simulink model "SF015A_WhlImbRejctn"  (R2013b)
settings: Solver=FixedStepDiscrete  SolverMode=SingleTasking  StartTime=0.0  StopTime=1  FixedStep=0.002  RelTol=1e-3
values from neighbouring files (symbols this model uses):
  ACTIVBANDMAX_ULS_U32 = DataDict.Constant    [SF015A_WhlImbRejctn_DataDict.m]
  ADAPVFILMAX_ULS_F32 = DataDict.Constant    [SF015A_WhlImbRejctn_DataDict.m]
  ARCHGLBPRM_180OVERPI_ULS_F32 = DataDict.Constant    [SF015A_WhlImbRejctn_DataDict.m]
  ARCHGLBPRM_2MILLISEC_SEC_F32 = DataDict.Constant    [SF015A_WhlImbRejctn_DataDict.m]
  ARCHGLBPRM_2PI_ULS_F32 = DataDict.Constant    [SF015A_WhlImbRejctn_DataDict.m]
  ARCHGLBPRM_FLOATZEROTHD_ULS_F32 = DataDict.Constant    [SF015A_WhlImbRejctn_DataDict.m]
  ARCHGLBPRM_PI_ULS_F32 = DataDict.Constant    [SF015A_WhlImbRejctn_DataDict.m]
  ARCHGLBPRM_PIOVER180_ULS_F32 = DataDict.Constant    [SF015A_WhlImbRejctn_DataDict.m]
  ARCHGLBPRM_PIOVER2_ULS_F32 = DataDict.Constant    [SF015A_WhlImbRejctn_DataDict.m]
  CALMINSPERCOUNT_ULS_F32 = DataDict.Constant    [SF015A_WhlImbRejctn_DataDict.m]
  DURATIONDISABLE_CNT_U16 = DataDict.Constant    [SF015A_WhlImbRejctn_DataDict.m]
  FILTWHLSPDMAX_MOTRADPERSEC_F32 = DataDict.Constant    [SF015A_WhlImbRejctn_DataDict.m]
  MICROSECTOMILLISEC_ULS_F32 = DataDict.Constant    [SF015A_WhlImbRejctn_DataDict.m]
  MINSTOMILLISEC_ULS_F32 = DataDict.Constant    [SF015A_WhlImbRejctn_DataDict.m]
  NINETY_ULS_F32 = DataDict.Constant    [SF015A_WhlImbRejctn_DataDict.m]
  NODEBSTEP_CNT_U16 = DataDict.Constant    [SF015A_WhlImbRejctn_DataDict.m]
  NROFDLY_CNT_U08 = DataDict.Constant    [SF015A_WhlImbRejctn_DataDict.m]
  ONEHALF_ULS_F32 = DataDict.Constant    [SF015A_WhlImbRejctn_DataDict.m]
  ONEHUNDRED_ULS_F32 = DataDict.Constant    [SF015A_WhlImbRejctn_DataDict.m]
  ONEOVRTHREE_ULS_F32 = DataDict.Constant    [SF015A_WhlImbRejctn_DataDict.m]
  ONEOVRTWENTY_ULS_F32 = DataDict.Constant    [SF015A_WhlImbRejctn_DataDict.m]
  ONETHOUSAND_ULS_F32 = DataDict.Constant    [SF015A_WhlImbRejctn_DataDict.m]
  PEAKMAX_ULS_F32 = DataDict.Constant    [SF015A_WhlImbRejctn_DataDict.m]
  PEAKMIN_ULS_F32 = DataDict.Constant    [SF015A_WhlImbRejctn_DataDict.m]
  PHAADJMAX_ULS_F32 = DataDict.Constant    [SF015A_WhlImbRejctn_DataDict.m]
  PITIMESSAMPLETIME_ULS_F32 = DataDict.Constant    [SF015A_WhlImbRejctn_DataDict.m]
  STOREDMINSPERCOUNT_ULS_F32 = DataDict.Constant    [SF015A_WhlImbRejctn_DataDict.m]
  TWO_ULS_F32 = DataDict.Constant    [SF015A_WhlImbRejctn_DataDict.m]
  TWOOVRTHREE_ULS_F32 = DataDict.Constant    [SF015A_WhlImbRejctn_DataDict.m]
  WhlImbRejctnAdpvFac = DataDict.Calibration    [SF015A_WhlImbRejctn_DataDict.m]
  WhlImbRejctnAutScaEna = DataDict.Calibration    [SF015A_WhlImbRejctn_DataDict.m]
  WhlImbRejctnAutScaTar = DataDict.Calibration    [SF015A_WhlImbRejctn_DataDict.m]
  WhlImbRejctnCurrMgnSlewPerLoop = DataDict.Calibration    [SF015A_WhlImbRejctn_DataDict.m]
  WhlImbRejctnDcTrendFltRcvryDly = DataDict.Calibration    [SF015A_WhlImbRejctn_DataDict.m]
  WhlImbRejctnDcTrendFltRcvryNegStep = DataDict.Calibration    [SF015A_WhlImbRejctn_DataDict.m]
  WhlImbRejctnDcTrendFltRcvryPosStep = DataDict.Calibration    [SF015A_WhlImbRejctn_DataDict.m]
  WhlImbRejctnDcTrendFltRcvryThd = DataDict.Calibration    [SF015A_WhlImbRejctn_DataDict.m]
  WhlImbRejctnDcTrendTh2Tq = DataDict.Calibration    [SF015A_WhlImbRejctn_DataDict.m]
  WhlImbRejctnDcTrendThTq = DataDict.Calibration    [SF015A_WhlImbRejctn_DataDict.m]
  WhlImbRejctnDcTrendTi2Sec = DataDict.Calibration    [SF015A_WhlImbRejctn_DataDict.m]
  WhlImbRejctnDcTrendTiSec = DataDict.Calibration    [SF015A_WhlImbRejctn_DataDict.m]
  WhlImbRejctnEnaSlewPerLoop = DataDict.Calibration    [SF015A_WhlImbRejctn_DataDict.m]
  WhlImbRejctnFctEna = DataDict.Calibration    [SF015A_WhlImbRejctn_DataDict.m]
  WhlImbRejctnFrqDiagcAmpThd = DataDict.Calibration    [SF015A_WhlImbRejctn_DataDict.m]
  WhlImbRejctnFrqDiagcEna = DataDict.Calibration    [SF015A_WhlImbRejctn_DataDict.m]
  WhlImbRejctnFrqDiagcFltRcvryDly = DataDict.Calibration    [SF015A_WhlImbRejctn_DataDict.m]
  WhlImbRejctnFrqDiagcFltRcvryNegStep = DataDict.Calibration    [SF015A_WhlImbRejctn_DataDict.m]
  WhlImbRejctnFrqDiagcFltRcvryPosStep = DataDict.Calibration    [SF015A_WhlImbRejctn_DataDict.m]
  WhlImbRejctnFrqDiagcFltRcvryThd = DataDict.Calibration    [SF015A_WhlImbRejctn_DataDict.m]
  WhlImbRejctnFrqDiagcThd = DataDict.Calibration    [SF015A_WhlImbRejctn_DataDict.m]
  WhlImbRejctnFrqDiagcTout = DataDict.Calibration    [SF015A_WhlImbRejctn_DataDict.m]
  WhlImbRejctnFrqDiagcUgrPoleMgn = DataDict.Calibration    [SF015A_WhlImbRejctn_DataDict.m]
  WhlImbRejctnFrqScaTblX = DataDict.Calibration    [SF015A_WhlImbRejctn_DataDict.m]
  WhlImbRejctnMaxDurn = DataDict.Calibration    [SF015A_WhlImbRejctn_DataDict.m]
  WhlImbRejctnMaxMgn = DataDict.Calibration    [SF015A_WhlImbRejctn_DataDict.m]
  WhlImbRejctnMaxMgnFltNegStep = DataDict.Calibration    [SF015A_WhlImbRejctn_DataDict.m]
  WhlImbRejctnMaxMgnFltPosStep = DataDict.Calibration    [SF015A_WhlImbRejctn_DataDict.m]
  WhlImbRejctnMaxMgnFltRcvryDly = DataDict.Calibration    [SF015A_WhlImbRejctn_DataDict.m]
  WhlImbRejctnMaxMgnFltRcvryNegStep = DataDict.Calibration    [SF015A_WhlImbRejctn_DataDict.m]
  WhlImbRejctnMaxMgnFltRcvryPosStep = DataDict.Calibration    [SF015A_WhlImbRejctn_DataDict.m]
  WhlImbRejctnMaxMgnFltRcvryThd = DataDict.Calibration    [SF015A_WhlImbRejctn_DataDict.m]
  WhlImbRejctnMaxMgnFltThd = DataDict.Calibration    [SF015A_WhlImbRejctn_DataDict.m]
  WhlImbRejctnMgnEstimnDeltaSca = DataDict.Calibration    [SF015A_WhlImbRejctn_DataDict.m]
  WhlImbRejctnMgnEstimnDiThd = DataDict.Calibration    [SF015A_WhlImbRejctn_DataDict.m]
  WhlImbRejctnMgnEstimnEnaThd = DataDict.Calibration    [SF015A_WhlImbRejctn_DataDict.m]
  WhlImbRejctnMgnEstimnFrq = DataDict.Calibration    [SF015A_WhlImbRejctn_DataDict.m]
  WhlImbRejctnMgnEstimnFrqDelta = DataDict.Calibration    [SF015A_WhlImbRejctn_DataDict.m]
  WhlImbRejctnMgnEstimnLeak = DataDict.Calibration    [SF015A_WhlImbRejctn_DataDict.m]
  WhlImbRejctnRampDwnTi = DataDict.Calibration    [SF015A_WhlImbRejctn_DataDict.m]
  WhlImbRejctnScaCncl = DataDict.Calibration    [SF015A_WhlImbRejctn_DataDict.m]
  WhlImbRejctnUgrPoleMgn = DataDict.Calibration    [SF015A_WhlImbRejctn_DataDict.m]
  WhlImbRejctnVehSpdEna = DataDict.Calibration    [SF015A_WhlImbRejctn_DataDict.m]
  WhlImbRejctnWhlSpdCorrlnFltRcvryDly = DataDict.Calibration    [SF015A_WhlImbRejctn_DataDict.m]
  WhlImbRejctnWhlSpdCorrlnFltRcvryNegStep = DataDict.Calibration    [SF015A_WhlImbRejctn_DataDict.m]
  WhlImbRejctnWhlSpdCorrlnFltRcvryPosStep = DataDict.Calibration    [SF015A_WhlImbRejctn_DataDict.m]
  WhlImbRejctnWhlSpdCorrlnFltRcvryThd = DataDict.Calibration    [SF015A_WhlImbRejctn_DataDict.m]
  WhlImbRejctnWhlSpdCorrlnThd = DataDict.Calibration    [SF015A_WhlImbRejctn_DataDict.m]
  WhlImbRejctnWhlSpdCorrlnTi = DataDict.Calibration    [SF015A_WhlImbRejctn_DataDict.m]
  WIRCMDMAX_MOTNWTMTR_F32 = DataDict.Constant    [SF015A_WhlImbRejctn_DataDict.m]
  ZERO_ULS_F32 = DataDict.Constant    [SF015A_WhlImbRejctn_DataDict.m]
undefined symbols (not defined in the file or in its folder): Cntr, NtcNr1, NvmGetErrSts1, SigQlfr1, Sts, SysSt1
libraries: simulink x32, FixdToFloat x32, Fil x20, NxtrLim x15, NxtrNvM x12, NxtrAbslt x8, NxtrMath x7, NxtrMax x6, NxtrMin x4, FloatToFixd x2, LnrIntrpn x2, NxtrSign x1
(part 7 of 12)

== system SF015A_WhlImbRejctn/WhlImbRejctn/WhlImbRejctnPer1/WIR Diagnostics/DcTrendDiag/NoFault ==
  Input : Inport
  Action Port : ActionPort  ActionType=else
  CopyRight2 : Subsystem  Description=|  mask(Copyright Information){none=on}
      | Copyright info block.                                               
      |                                                                     
      | Place copyright information at the top of every subsystem in design.
      mask prompts: none "No parameters"
      mask help: Place copyright information at the top of every subsystem in design.
      mask Display:
      | NxtrConf = 'Nexteer Confidential';
      | 
      | sys = bdroot; %handle for the current model ("system")
      | first = get_param(sys,'Created');
      | if(isempty(first))
      |     first = datestr(now,'yyyy');
      | else
      |     first = first(end-3:end);  %year is last four digits
      | end
      | 
      | last = get_param(sys,'LastModifiedDate');
      | if isempty(last)
      |     last = datestr(now,'yyyy');
      | else
      |     last = last(end-3:end);
      | end
      | 
      | if strcmp(first,last)
      |     fprintf('%s -- Copyright %s Nexteer',NxtrConf,first)
      | else
      |     fprintf('%s -- %s%s- %s Nexteer',NxtrConf,char(169),first,last)
      | end
  Output : Outport
  wires:
  Input/1 -> Output/1

== system SF015A_WhlImbRejctn/WhlImbRejctn/WhlImbRejctnPer1/WIR Diagnostics/FrequencyDiag/CopyRight2 ==

== system SF015A_WhlImbRejctn/WhlImbRejctn/WhlImbRejctnPer1/WIR Diagnostics/FrequencyDiag/EnableDiag ==
  WIRCmdAmp : Inport
  FreqEst : Inport  Port=2
  WIRCmd : Inport  Port=3
  Enable : Inport  Port=4
  Action Port : ActionPort  ActionType=then
  CopyRight2 : Subsystem  Description=|  mask(Copyright Information){none=on}
      | Copyright info block.                                               
      |                                                                     
      | Place copyright information at the top of every subsystem in design.
      mask prompts: none "No parameters"
      mask help: Place copyright information at the top of every subsystem in design.
      mask Display:
      | NxtrConf = 'Nexteer Confidential';
      | 
      | sys = bdroot; %handle for the current model ("system")
      | first = get_param(sys,'Created');
      | if(isempty(first))
      |     first = datestr(now,'yyyy');
      | else
      |     first = first(end-3:end);  %year is last four digits
      | end
      | 
      | last = get_param(sys,'LastModifiedDate');
      | if isempty(last)
      |     last = datestr(now,'yyyy');
      | else
      |     last = last(end-3:end);
      | end
      | 
      | if strcmp(first,last)
      |     fprintf('%s -- Copyright %s Nexteer',NxtrConf,first)
      | else
      |     fprintf('%s -- %s%s- %s Nexteer',NxtrConf,char(169),first,last)
      | end
  Notch Comparison : Subsystem
  Output : Outport
  wires:
  Notch Comparison/1(FreqDiag) -> Output/1
  WIRCmdAmp/1 -> Notch Comparison/1(WIRCmdAmp)
  FreqEst/1 -> Notch Comparison/2(FreqEst)
  WIRCmd/1 -> Notch Comparison/3(WIRCmd)
  Enable/1 -> Notch Comparison/4(Enable)

== system SF015A_WhlImbRejctn/WhlImbRejctn/WhlImbRejctnPer1/WIR Diagnostics/FrequencyDiag/FreqDiagFault ==
  Input : Inport
  Action Port : ActionPort  ActionType=then
  CopyRight2 : Subsystem  Description=|  mask(Copyright Information){none=on}
      | Copyright info block.                                               
      |                                                                     
      | Place copyright information at the top of every subsystem in design.
      mask prompts: none "No parameters"
      mask help: Place copyright information at the top of every subsystem in design.
      mask Display:
      | NxtrConf = 'Nexteer Confidential';
      | 
      | sys = bdroot; %handle for the current model ("system")
      | first = get_param(sys,'Created');
      | if(isempty(first))
      |     first = datestr(now,'yyyy');
      | else
      |     first = first(end-3:end);  %year is last four digits
      | end
      | 
      | last = get_param(sys,'LastModifiedDate');
      | if isempty(last)
      |     last = datestr(now,'yyyy');
      | else
      |     last = last(end-3:end);
      | end
      | 
      | if strcmp(first,last)
      |     fprintf('%s -- Copyright %s Nexteer',NxtrConf,first)
      | else
      |     fprintf('%s -- %s%s- %s Nexteer',NxtrConf,char(169),first,last)
      | end
  Output : Outport
  wires:
  Input/1 -> Output/1

== system SF015A_WhlImbRejctn/WhlImbRejctn/WhlImbRejctnPer1/WIR Diagnostics/FrequencyDiag/NoDiag ==
  Input : Inport
  Action Port : ActionPort  ActionType=else
  CopyRight2 : Subsystem  Description=|  mask(Copyright Information){none=on}
      | Copyright info block.                                               
      |                                                                     
      | Place copyright information at the top of every subsystem in design.
      mask prompts: none "No parameters"
      mask help: Place copyright information at the top of every subsystem in design.
      mask Display:
      | NxtrConf = 'Nexteer Confidential';
      | 
      | sys = bdroot; %handle for the current model ("system")
      | first = get_param(sys,'Created');
      | if(isempty(first))
      |     first = datestr(now,'yyyy');
      | else
      |     first = first(end-3:end);  %year is last four digits
      | end
      | 
      | last = get_param(sys,'LastModifiedDate');
      | if isempty(last)
      |     last = datestr(now,'yyyy');
      | else
      |     last = last(end-3:end);
      | end
      | 
      | if strcmp(first,last)
      |     fprintf('%s -- Copyright %s Nexteer',NxtrConf,first)
      | else
      |     fprintf('%s -- %s%s- %s Nexteer',NxtrConf,char(169),first,last)
      | end
  Output : Outport
  wires:
  Input/1 -> Output/1

== system SF015A_WhlImbRejctn/WhlImbRejctn/WhlImbRejctnPer1/WIR Diagnostics/FrequencyDiag/NoFault ==
  Input : Inport
  Action Port : ActionPort  ActionType=else
  CopyRight2 : Subsystem  Description=|  mask(Copyright Information){none=on}
      | Copyright info block.                                               
      |                                                                     
      | Place copyright information at the top of every subsystem in design.
      mask prompts: none "No parameters"
      mask help: Place copyright information at the top of every subsystem in design.
      mask Display:
      | NxtrConf = 'Nexteer Confidential';
      | 
      | sys = bdroot; %handle for the current model ("system")
      | first = get_param(sys,'Created');
      | if(isempty(first))
      |     first = datestr(now,'yyyy');
      | else
      |     first = first(end-3:end);  %year is last four digits
      | end
      | 
      | last = get_param(sys,'LastModifiedDate');
      | if isempty(last)
      |     last = datestr(now,'yyyy');
      | else
      |     last = last(end-3:end);
      | end
      | 
      | if strcmp(first,last)
      |     fprintf('%s -- Copyright %s Nexteer',NxtrConf,first)
      | else
      |     fprintf('%s -- %s%s- %s Nexteer',NxtrConf,char(169),first,last)
      | end
  Output : Outport
  wires:
  Input/1 -> Output/1

== system SF015A_WhlImbRejctn/WhlImbRejctn/WhlImbRejctnPer1/WIR Diagnostics/MaxMagDiag/CopyRight2 ==

== system SF015A_WhlImbRejctn/WhlImbRejctn/WhlImbRejctnPer1/WIR Diagnostics/MaxMagDiag/Magnitude Comparison ==
  WIRCmdAmp1 : Inport
  Constant1 : Constant  Value=WhlImbRejctnMaxMgnFltPosStep
  Constant5 : Constant  Value=WhlImbRejctnMaxMgnFltNegStep
  Constant6 : Constant  Value=WhlImbRejctnMaxMgnFltThd
  Constant7 : Constant  Value=WhlImbRejctnMaxMgn
  CopyRight2 : Subsystem  Description=|  mask(Copyright Information){none=on}
      | Copyright info block.                                               
      |                                                                     
      | Place copyright information at the top of every subsystem in design.
      mask prompts: none "No parameters"
      mask help: Place copyright information at the top of every subsystem in design.
      mask Display:
      | NxtrConf = 'Nexteer Confidential';
      | 
      | sys = bdroot; %handle for the current model ("system")
      | first = get_param(sys,'Created');
      | first = first(end-3:end);  %year is last four digits
      | 
      | last = get_param(sys,'LastModifiedDate');
      | if isempty(last)
      |     last = datestr(now,'yyyy');
      | else
      |     last = last(end-3:end);
      | end
      | 
      | if strcmp(first,last)
      |     fprintf('%s -- Copyright %s Nexteer',NxtrConf,first)
      | else
      |     fprintf('%s -- %s%s- %s Nexteer',NxtrConf,char(169),first,last)
      | end
  Diagnostic Threshold : Subsystem
  Relational Operator2 : RelationalOperator  OutDataTypeStr=boolean
  MagDiag : Outport
  wires:
  Diagnostic Threshold/1(DiagFailed) -> MagDiag/1
  Constant1/1 -> Diagnostic Threshold/2(PStepIncrement)
  WIRCmdAmp1/1 -> Relational Operator2/1
  Constant7/1 -> Relational Operator2/2
  Relational Operator2/1 -> Diagnostic Threshold/1(Fault Present)
  Constant5/1 -> Diagnostic Threshold/3(NStepIncrement)
  Constant6/1 -> Diagnostic Threshold/4(Threshold)

== system SF015A_WhlImbRejctn/WhlImbRejctn/WhlImbRejctnPer1/WIR Diagnostics/Set NTC Block/CopyRight2 ==

== system SF015A_WhlImbRejctn/WhlImbRejctn/WhlImbRejctnPer1/WIR Diagnostics/Set NTC Block/NTC Bit parameter info ==
  Flag : Inport
  Constant10 : Constant  OutDataTypeStr=uint8
  Constant5 : Constant  Value=0  OutDataTypeStr=uint8
  If : If  IfExpression=u1
  If Action Subsystem : Subsystem  TreatAsAtomicUnit=on
  If Action Subsystem1 : Subsystem  TreatAsAtomicUnit=on
  Merge : Merge
  FltBit : Outport
  wires:
  Flag/1 -> If/1
  If/1 -> If Action Subsystem/Action
  Constant5/1 -> If Action Subsystem1/1(In1)
  If/2 -> If Action Subsystem1/Action
  Constant10/1 -> If Action Subsystem/1(In1)
  Merge/1 -> FltBit/1
  If Action Subsystem/1(Out1) -> Merge/1
  If Action Subsystem1/1(Out1) -> Merge/2

== system SF015A_WhlImbRejctn/WhlImbRejctn/WhlImbRejctnPer1/WIR Diagnostics/Set NTC Block/NTC Bit parameter info2 ==
  Flag : Inport
  Constant10 : Constant  Value=4  OutDataTypeStr=uint8
  Constant5 : Constant  Value=0  OutDataTypeStr=uint8
  If : If  IfExpression=u1
  If Action Subsystem : Subsystem  TreatAsAtomicUnit=on
  If Action Subsystem1 : Subsystem  TreatAsAtomicUnit=on
  Merge : Merge
  FltBit : Outport
  wires:
  Flag/1 -> If/1
  If/1 -> If Action Subsystem/Action
  Constant5/1 -> If Action Subsystem1/1(In1)
  If/2 -> If Action Subsystem1/Action
  Constant10/1 -> If Action Subsystem/1(In1)
  Merge/1 -> FltBit/1
  If Action Subsystem/1(Out1) -> Merge/1
  If Action Subsystem1/1(Out1) -> Merge/2

== system SF015A_WhlImbRejctn/WhlImbRejctn/WhlImbRejctnPer1/WIR Diagnostics/Set NTC Block/NTC Bit parameter info3 ==
  Flag : Inport
  Constant10 : Constant  Value=8  OutDataTypeStr=uint8
  Constant5 : Constant  Value=0  OutDataTypeStr=uint8
  If : If  IfExpression=u1
  If Action Subsystem : Subsystem  TreatAsAtomicUnit=on
  If Action Subsystem1 : Subsystem  TreatAsAtomicUnit=on
  Merge : Merge
  FltBit : Outport
  wires:
  Flag/1 -> If/1
  If/1 -> If Action Subsystem/Action
  Constant5/1 -> If Action Subsystem1/1(In1)
  If/2 -> If Action Subsystem1/Action
  Constant10/1 -> If Action Subsystem/1(In1)
  Merge/1 -> FltBit/1
  If Action Subsystem/1(Out1) -> Merge/1
  If Action Subsystem1/1(Out1) -> Merge/2

== system SF015A_WhlImbRejctn/WhlImbRejctn/WhlImbRejctnPer1/WIR Diagnostics/Set NTC Block/NTC Bit parameter info4 ==
  Flag : Inport
  Constant10 : Constant  Value=16  OutDataTypeStr=uint8
  Constant5 : Constant  Value=0  OutDataTypeStr=uint8
  If : If  IfExpression=u1
  If Action Subsystem : Subsystem  TreatAsAtomicUnit=on
  If Action Subsystem1 : Subsystem  TreatAsAtomicUnit=on
  Merge : Merge
  FltBit : Outport
  wires:
  Flag/1 -> If/1
  If/1 -> If Action Subsystem/Action
  Constant5/1 -> If Action Subsystem1/1(In1)
  If/2 -> If Action Subsystem1/Action
  Constant10/1 -> If Action Subsystem/1(In1)
  Merge/1 -> FltBit/1
  If Action Subsystem/1(Out1) -> Merge/1
  If Action Subsystem1/1(Out1) -> Merge/2

== system SF015A_WhlImbRejctn/WhlImbRejctn/WhlImbRejctnPer1/WIR Diagnostics/Set NTC Block/NTC Bit parameter info5 ==
  Flag : Inport
  Constant10 : Constant  Value=32  OutDataTypeStr=uint8
  Constant5 : Constant  Value=0  OutDataTypeStr=uint8
  If : If  IfExpression=u1
  If Action Subsystem : Subsystem  TreatAsAtomicUnit=on
  If Action Subsystem1 : Subsystem  TreatAsAtomicUnit=on
  Merge : Merge
  FltBit : Outport
  wires:
  Flag/1 -> If/1
  If/1 -> If Action Subsystem/Action
  Constant5/1 -> If Action Subsystem1/1(In1)
  If/2 -> If Action Subsystem1/Action
  Constant10/1 -> If Action Subsystem/1(In1)
  Merge/1 -> FltBit/1
  If Action Subsystem/1(Out1) -> Merge/1
  If Action Subsystem1/1(Out1) -> Merge/2

== system SF015A_WhlImbRejctn/WhlImbRejctn/WhlImbRejctnPer1/WIR Diagnostics/Set NTC Block/SetNtcSts ==
  note: Note:
      |
      | - "ISO Fault Debounce Design" Simulink block intent to use here for Simulation purpose only. Do not Code this block
  NtcNr : Inport
  NtcStInfo : Inport  Port=2
  NtcSts : Inport  Port=3
  DebStep : Inport  Port=4
  CopyRight2 : Subsystem  Description=|  mask(Copyright Information){none=on}
      | Copyright info block.                                               
      |                                                                     
      | Place copyright information at the top of every subsystem in design.
      mask prompts: none "No parameters"
      mask help: Place copyright information at the top of every subsystem in design.
      mask Display:
      | NxtrConf = 'Nexteer Confidential';
      | 
      | sys = bdroot; %handle for the current model ("system")
      | first = get_param(sys,'Created');
      | first = first(end-3:end);  %year is last four digits
      | 
      | last = get_param(sys,'LastModifiedDate');
      | if isempty(last)
      |     last = datestr(now,'yyyy');
      | else
      |     last = last(end-3:end);
      | end
      | 
      | if strcmp(first,last)
      |     fprintf('%s -- Copyright %s Nexteer',NxtrConf,first)
      | else
      |     fprintf('%s -- %s%s- %s Nexteer',NxtrConf,char(169),first,last)
      | end
  Data Store Write : DataStoreWrite  Commented=on  DataStoreName=NtcQlfr
  Ground : Ground  Commented=on
  ISO Fault Debounce Design : Subsystem  Commented=on  TreatAsAtomicUnit=on
      settings: AttributesFormatString=|
      | Simulation Purpose Only.
      | Do Not Code this block
      | Diagnostic Manager Owns this requirement
  Terminator{,1..3} (4 alike) : Terminator
  wires:
  NtcStInfo/1 -> Terminator1/1
  NtcNr/1 -> Terminator/1
  NtcSts/1 -> Terminator2/1
  DebStep/1 -> Terminator3/1
  ISO Fault Debounce Design/1(Qualifier) -> Data Store Write/1
  Ground/1 -> ISO Fault Debounce Design/3(SvcClr)

== system SF015A_WhlImbRejctn/WhlImbRejctn/WhlImbRejctnPer1/WIR Diagnostics/WhlSpdCorrDiag/CopyRight2 ==

== system SF015A_WhlImbRejctn/WhlImbRejctn/WhlImbRejctnPer1/WIR Diagnostics/WhlSpdCorrDiag/ElapsedTime1 ==
  FltStsTrue : Inport
  Data Store Read : DataStoreRead  Priority=1  DataStoreName=WhlSpdCorrlnLrngEnaPrevTmr
      settings: AttributesFormatString="priority:  %<Priority>"
  Data Store Write : DataStoreWrite  Priority=2  DataStoreName=WhlSpdCorrlnLrngEnaPrevTmr
      settings: AttributesFormatString="priority:  %<Priority>"
  If : If  NumInputs=2  IfExpression=u1  ElseIfExpressions=u2
  If not true elapsed time = 0 : Subsystem  TreatAsAtomicUnit=on
  "If true and last step is true calculate elapsed time " : Subsystem  TreatAsAtomicUnit=on
  "If true and last step not true elapsed time = 0 get reference time " : Subsystem  TreatAsAtomicUnit=on
  Logical Operator1 : Logic  Operator=NOT  AllPortsSameDT=off  OutDataTypeStr=boolean
  Logical Operator2 : Logic  Operator=NOT  AllPortsSameDT=off  OutDataTypeStr=boolean
  Merge : Merge  Inputs=3
  ElapsedTime : Outport
  wires:
  If/1 -> If not true elapsed time = 0/Action
  If/2 -> "If true and last step not true elapsed time = 0 get reference time "/Action
  If/3 -> "If true and last step is true calculate elapsed time "/Action
  If not true elapsed time = 0/1(SpanTi) -> Merge/1
  "If true and last step not true elapsed time = 0 get reference time "/1("SpanTi ") -> Merge/2
  "If true and last step is true calculate elapsed time "/1(SpanTi) -> Merge/3
  Merge/1 -> ElapsedTime/1
  FltStsTrue/1 -> Logical Operator2/1, Data Store Write/1
  Data Store Read/1 -> Logical Operator1/1
  Logical Operator2/1 -> If/1
  Logical Operator1/1 -> If/2

== system SF015A_WhlImbRejctn/WhlImbRejctn/WhlImbRejctnPer1/WIR Diagnostics/WhlSpdCorrDiag/FullCrrln ==
  Input : Inport
  Action Port : ActionPort  ActionType=then
  CopyRight2 : Subsystem  Description=|  mask(Copyright Information){none=on}
      | Copyright info block.                                               
      |                                                                     
      | Place copyright information at the top of every subsystem in design.
      mask prompts: none "No parameters"
      mask help: Place copyright information at the top of every subsystem in design.
      mask Display:
      | NxtrConf = 'Nexteer Confidential';
      | 
      | sys = bdroot; %handle for the current model ("system")
      | first = get_param(sys,'Created');
      | if(isempty(first))
      |     first = datestr(now,'yyyy');
      | else
      |     first = first(end-3:end);  %year is last four digits
      | end
      | 
      | last = get_param(sys,'LastModifiedDate');
      | if isempty(last)
      |     last = datestr(now,'yyyy');
      | else
      |     last = last(end-3:end);
      | end
      | 
      | if strcmp(first,last)
      |     fprintf('%s -- Copyright %s Nexteer',NxtrConf,first)
      | else
      |     fprintf('%s -- %s%s- %s Nexteer',NxtrConf,char(169),first,last)
      | end
  Output : Outport
  wires:
  Input/1 -> Output/1

== system SF015A_WhlImbRejctn/WhlImbRejctn/WhlImbRejctnPer1/WIR Diagnostics/WhlSpdCorrDiag/NoFault ==
  Input : Inport
  Action Port : ActionPort  ActionType=else
  CopyRight2 : Subsystem  Description=|  mask(Copyright Information){none=on}
      | Copyright info block.                                               
      |                                                                     
      | Place copyright information at the top of every subsystem in design.
      mask prompts: none "No parameters"
      mask help: Place copyright information at the top of every subsystem in design.
      mask Display:
      | NxtrConf = 'Nexteer Confidential';
      | 
      | sys = bdroot; %handle for the current model ("system")
      | first = get_param(sys,'Created');
      | if(isempty(first))
      |     first = datestr(now,'yyyy');
      | else
      |     first = first(end-3:end);  %year is last four digits
      | end
      | 
      | last = get_param(sys,'LastModifiedDate');
      | if isempty(last)
      |     last = datestr(now,'yyyy');
      | else
      |     last = last(end-3:end);
      | end
      | 
      | if strcmp(first,last)
      |     fprintf('%s -- Copyright %s Nexteer',NxtrConf,first)
      | else
      |     fprintf('%s -- %s%s- %s Nexteer',NxtrConf,char(169),first,last)
      | end
  Output : Outport
  wires:
  Input/1 -> Output/1

== system SF015A_WhlImbRejctn/WhlImbRejctn/WhlImbRejctnPer1/WIR Diagnostics/WhlSpdCorrDiag/WhlFreq In Range ==
  WhlFreq : Inport
  Add : Sum  Inputs=+-
  Constant1 : Constant
  Constant2 : Constant  Value=WhlImbRejctnFrqScaTblX
  Constant3 : Constant  Value=WhlImbRejctnFrqScaTblX
  Constant4 : Constant  Value=0
  FixdToFloat_f32_u1 : FixdToFloat/FixdToFloat_f32_u16  Param1=0
  FixdToFloat_f32_u16 : FixdToFloat/FixdToFloat_f32_u16  Param1=0
  Logical Operator1 : Logic  AllPortsSameDT=off  OutDataTypeStr=boolean
  Relational Operator1 : RelationalOperator  Operator=<=  OutDataTypeStr=boolean
  Relational Operator2 : RelationalOperator  OutDataTypeStr=boolean
  Selector3 : Selector  IndexMode=Zero-based  InputPortWidth=6  IndexOptions=Index vector (port)  Indices=[1]  OutputSizes=1
  Selector4 : Selector  IndexMode=Zero-based  InputPortWidth=6  IndexOptions=Index vector (port)  Indices=[1]  OutputSizes=1
  Width : Width
  InRng : Outport
  wires:
  WhlFreq/1 -> Relational Operator2/1, Relational Operator1/1
  Relational Operator2/1 -> Logical Operator1/1
  Relational Operator1/1 -> Logical Operator1/2
  Logical Operator1/1 -> InRng/1
  FixdToFloat_f32_u16/1 -> Relational Operator2/2
  FixdToFloat_f32_u1/1 -> Relational Operator1/2
  Selector3/1 -> FixdToFloat_f32_u1/1
  Selector4/1 -> FixdToFloat_f32_u16/1
  Constant3/1 -> Width/1, Selector3/1
  Constant4/1 -> Selector4/2
  Width/1 -> Add/1
  Add/1 -> Selector3/2
  Constant1/1 -> Add/2
  Constant2/1 -> Selector4/1

== system SF015A_WhlImbRejctn/WhlImbRejctn/WhlImbRejctnPer1/WIR Diagnostics/WhlSpdCorrDiag/WhlFreq In Range1 ==
  WhlFreq : Inport
  Add : Sum  Inputs=+-
  Constant1 : Constant
  Constant2 : Constant  Value=WhlImbRejctnFrqScaTblX
  Constant3 : Constant  Value=WhlImbRejctnFrqScaTblX
  Constant4 : Constant  Value=0
  FixdToFloat_f32_u1 : FixdToFloat/FixdToFloat_f32_u16  Param1=0
  FixdToFloat_f32_u16 : FixdToFloat/FixdToFloat_f32_u16  Param1=0
  Logical Operator1 : Logic  AllPortsSameDT=off  OutDataTypeStr=boolean
  Relational Operator1 : RelationalOperator  Operator=<=  OutDataTypeStr=boolean
  Relational Operator2 : RelationalOperator  OutDataTypeStr=boolean
  Selector3 : Selector  IndexMode=Zero-based  InputPortWidth=6  IndexOptions=Index vector (port)  Indices=[1]  OutputSizes=1
  Selector4 : Selector  IndexMode=Zero-based  InputPortWidth=6  IndexOptions=Index vector (port)  Indices=[1]  OutputSizes=1
  Width : Width
  InRng : Outport
  wires:
  WhlFreq/1 -> Relational Operator2/1, Relational Operator1/1
  Relational Operator2/1 -> Logical Operator1/1
  Relational Operator1/1 -> Logical Operator1/2
  Logical Operator1/1 -> InRng/1
  FixdToFloat_f32_u16/1 -> Relational Operator2/2
  FixdToFloat_f32_u1/1 -> Relational Operator1/2
  Selector3/1 -> FixdToFloat_f32_u1/1
  Selector4/1 -> FixdToFloat_f32_u16/1
  Constant3/1 -> Width/1, Selector3/1
  Constant4/1 -> Selector4/2
  Width/1 -> Add/1
  Add/1 -> Selector3/2
  Constant1/1 -> Add/2
  Constant2/1 -> Selector4/1

== system SF015A_WhlImbRejctn/WhlImbRejctn/WhlImbRejctnPer1/WIR Diagnostics/WhlSpdCorrDiag/WhlSpdFault ==
  Input : Inport
  Action Port : ActionPort  ActionType=then
  CopyRight2 : Subsystem  Description=|  mask(Copyright Information){none=on}
      | Copyright info block.                                               
      |                                                                     
      | Place copyright information at the top of every subsystem in design.
      mask prompts: none "No parameters"
      mask help: Place copyright information at the top of every subsystem in design.
      mask Display:
      | NxtrConf = 'Nexteer Confidential';
      | 
      | sys = bdroot; %handle for the current model ("system")
      | first = get_param(sys,'Created');
      | if(isempty(first))
      |     first = datestr(now,'yyyy');
      | else
      |     first = first(end-3:end);  %year is last four digits
      | end
      | 
      | last = get_param(sys,'LastModifiedDate');
      | if isempty(last)
      |     last = datestr(now,'yyyy');
      | else
      |     last = last(end-3:end);
      | end
      | 
      | if strcmp(first,last)
      |     fprintf('%s -- Copyright %s Nexteer',NxtrConf,first)
      | else
      |     fprintf('%s -- %s%s- %s Nexteer',NxtrConf,char(169),first,last)
      | end
  Output : Outport
  wires:
  Input/1 -> Output/1

== system SF015A_WhlImbRejctn/WhlImbRejctn/WhlImbRejctnPer1/WIR Diagnostics/WhlSpdCorrDiag/WhlSpdbasedCrrln ==
  Right : Inport
  Left : Inport  Port=2
  Action Port : ActionPort  ActionType=else
  Constant1 : Constant  Value=ONEHUNDRED_ULS_F32
  CopyRight2 : Subsystem  Description=|  mask(Copyright Information){none=on}
      | Copyright info block.                                               
      |                                                                     
      | Place copyright information at the top of every subsystem in design.
      mask prompts: none "No parameters"
      mask help: Place copyright information at the top of every subsystem in design.
      mask Display:
      | NxtrConf = 'Nexteer Confidential';
      | 
      | sys = bdroot; %handle for the current model ("system")
      | first = get_param(sys,'Created');
      | if(isempty(first))
      |     first = datestr(now,'yyyy');
      | else
      |     first = first(end-3:end);  %year is last four digits
      | end
      | 
      | last = get_param(sys,'LastModifiedDate');
      | if isempty(last)
      |     last = datestr(now,'yyyy');
      | else
      |     last = last(end-3:end);
      | end
      | 
      | if strcmp(first,last)
      |     fprintf('%s -- Copyright %s Nexteer',NxtrConf,first)
      | else
      |     fprintf('%s -- %s%s- %s Nexteer',NxtrConf,char(169),first,last)
      | end
  If2 : If  RequirementInfo={} %GIDa_0c0aa31b_11fe_4581_a810_3d460bb4db41  IfExpression=u1
  Merge1 : Merge
  No : Subsystem  RequirementInfo={} %GIDa_64a328b2_0a29_4cbd_b70d_eb89b2045f04  TreatAsAtomicUnit=on
  Product : Product  RndMeth=Zero
  Relational Operator2 : RelationalOperator  OutDataTypeStr=boolean
  Yes : Subsystem  RequirementInfo={} %GIDa_acf7a133_1f67_4b0f_a68e_7f54b12dfd9b  TreatAsAtomicUnit=on
  Output : Outport
  wires:
  Merge1/1 -> Product/1
  Constant1/1 -> Product/2
  Product/1 -> Output/1
  Right/1 -> [Right]
  If2/1 -> Yes/Action
  If2/2 -> No/Action
  Yes/1(Output) -> Merge1/1
  No/1(Output) -> Merge1/2
  Relational Operator2/1 -> If2/1
  Left/1 -> [Left]
  [Right] -> Relational Operator2/1
  [Left] -> Relational Operator2/2
  [Right] -> Yes/1(Right)
  [Left] -> Yes/2(Left)
  [Right] -> No/1(Right)
  [Left] -> No/2(Left)

== system SF015A_WhlImbRejctn/WhlImbRejctn/WhlImbRejctnPer1/Whl Spd filter and Freq Estimation/Tapped Delay Implementation/CopyRight2 ==

== system SF015A_WhlImbRejctn/WhlImbRejctn/WhlImbRejctnPer1/Whl Spd filter and Freq Estimation/Tapped Delay Implementation/If Action Subsystem ==
  Action Port : ActionPort  ActionType=then
  Constant : Constant  Value=0  OutDataTypeStr=uint8
  Out1 : Outport
  wires:
  Constant/1 -> Out1/1

== system SF015A_WhlImbRejctn/WhlImbRejctn/WhlImbRejctnPer1/Whl Spd filter and Freq Estimation/Tapped Delay Implementation/If Action Subsystem1 ==
  In1 : Inport
  Action Port : ActionPort  ActionType=else
  Out1 : Outport
  wires:
  In1/1 -> Out1/1

== system SF015A_WhlImbRejctn/WhlImbRejctn/WhlImbRejctnPer1/Whl Spd filter and Freq Estimation/Tapped Delay Implementation1/CopyRight2 ==

== system SF015A_WhlImbRejctn/WhlImbRejctn/WhlImbRejctnPer1/Whl Spd filter and Freq Estimation/Tapped Delay Implementation1/If Action Subsystem ==
  Action Port : ActionPort  ActionType=then
  Constant : Constant  Value=0  OutDataTypeStr=uint8
  Out1 : Outport
  wires:
  Constant/1 -> Out1/1

== system SF015A_WhlImbRejctn/WhlImbRejctn/WhlImbRejctnPer1/Whl Spd filter and Freq Estimation/Tapped Delay Implementation1/If Action Subsystem1 ==
  In1 : Inport
  Action Port : ActionPort  ActionType=else
  Out1 : Outport
  wires:
  In1/1 -> Out1/1

== system SF015A_WhlImbRejctn/WhlImbRejctn/WhlImbRejctnPer1/Whl Spd filter and Freq Estimation/UGR L/Calc_ma1_a2 ==
  note: Limit f_est to first and last
      | value in t_FreqScaleTblX
  f_est : Inport
  PoleMag : Inport  Port=2
  Add : Sum  Inputs=+-
  Constant1 : Constant
  Constant2 : Constant  Value=WhlImbRejctnFrqScaTblX
  Constant3 : Constant  Value=TWO_ULS_F32  OutDataTypeStr=single
  Constant4 : Constant  Value=WhlImbRejctnFrqScaTblX
  Constant5 : Constant  Value=0
  CopyRight2 : Subsystem  Description=|  mask(Copyright Information){none=on}
      | Copyright info block.                                               
      |                                                                     
      | Place copyright information at the top of every subsystem in design.
      mask prompts: none "No parameters"
      mask help: Place copyright information at the top of every subsystem in design.
      mask Display:
      | NxtrConf = 'Nexteer Confidential';
      | 
      | sys = bdroot; %handle for the current model ("system")
      | first = get_param(sys,'Created');
      | first = first(end-3:end);  %year is last four digits
      | 
      | last = get_param(sys,'LastModifiedDate');
      | if isempty(last)
      |     last = datestr(now,'yyyy');
      | else
      |     last = last(end-3:end);
      | end
      | 
      | if strcmp(first,last)
      |     fprintf('%s -- Copyright %s Nexteer',NxtrConf,first)
      | else
      |     fprintf('%s -- %s%s- %s Nexteer',NxtrConf,char(169),first,last)
      | end
  Cos_f32 : NxtrMath/Cos_f32  SFunctionSpec=single y1 = Cos_f32(single u1)
      settings: AttributesFormatString=%<MaskType>
  FixdToFloat_f32_u1 : FixdToFloat/FixdToFloat_f32_u16  Param1=0
  FixdToFloat_f32_u16 : FixdToFloat/FixdToFloat_f32_u16  Param1=0
  Gain : Gain  Gain=ARCHGLBPRM_2PI_ULS_F32
  LimDyn_f32 : NxtrLim/LimDyn_f32
  Math Function1 : Math  Operator=square  SaturateOnIntegerOverflow=on  OutDataTypeStr=Inherit: Inherit via internal rule
  Product1 : Product  Inputs=3  SaturateOnIntegerOverflow=on
  Product3 : Product  SaturateOnIntegerOverflow=on
  Selector3 : Selector  IndexMode=Zero-based  InputPortWidth=6  IndexOptions=Index vector (port)  Indices=[1]  OutputSizes=1
  Selector4 : Selector  IndexMode=Zero-based  InputPortWidth=6  IndexOptions=Index vector (port)  Indices=[1]  OutputSizes=1
  Ts : Constant  Value=ARCHGLBPRM_2MILLISEC_SEC_F32
  Width : Width
  minus_a1 : Outport
  a2 : Outport  Port=2
  wires:
  Gain/1 -> Cos_f32/1
  Product1/1 -> minus_a1/1  "ma1"
  Constant3/1 -> Product1/2
  Cos_f32/1 -> Product1/1
  Product3/1 -> Gain/1
  Ts/1 -> Product3/2
  PoleMag/1 -> Product1/3, Math Function1/1
  Math Function1/1 -> a2/1
  LimDyn_f32/1 -> Product3/1
  f_est/1 -> LimDyn_f32/1
  FixdToFloat_f32_u16/1 -> LimDyn_f32/3
  FixdToFloat_f32_u1/1 -> LimDyn_f32/2
  Selector3/1 -> FixdToFloat_f32_u16/1
  Selector4/1 -> FixdToFloat_f32_u1/1
  Constant4/1 -> Width/1, Selector3/1
  Constant5/1 -> Selector4/2
  Width/1 -> Add/1
  Add/1 -> Selector3/2
  Constant1/1 -> Add/2
  Constant2/1 -> Selector4/1

== system SF015A_WhlImbRejctn/WhlImbRejctn/WhlImbRejctnPer1/Whl Spd filter and Freq Estimation/UGR L/CopyRight2 ==

== system SF015A_WhlImbRejctn/WhlImbRejctn/WhlImbRejctnPer1/Whl Spd filter and Freq Estimation/UGR L/UnityGainResFilt ==
  y : Inport
  minus_a1 : Inport  Port=2
  a2 : Inport  Port=3
  Constant3 : Constant  Value=ONEHALF_ULS_F32
  CopyRight2 : Subsystem  Description=|  mask(Copyright Information){none=on}
      | Copyright info block.                                               
      |                                                                     
      | Place copyright information at the top of every subsystem in design.
      mask prompts: none "No parameters"
      mask help: Place copyright information at the top of every subsystem in design.
      mask Display:
      | NxtrConf = 'Nexteer Confidential';
      | 
      | sys = bdroot; %handle for the current model ("system")
      | first = get_param(sys,'Created');
      | first = first(end-3:end);  %year is last four digits
      | 
      | last = get_param(sys,'LastModifiedDate');
      | if isempty(last)
      |     last = datestr(now,'yyyy');
      | else
      |     last = last(end-3:end);
      | end
      | 
      | if strcmp(first,last)
      |     fprintf('%s -- Copyright %s Nexteer',NxtrConf,first)
      | else
      |     fprintf('%s -- %s%s- %s Nexteer',NxtrConf,char(169),first,last)
      | end
  Data Store Read : DataStoreRead  Priority=1  DataStoreName=UgrLe2
      settings: AttributesFormatString=%<Priority>
  Data Store Read1 : DataStoreRead  Priority=1  DataStoreName=UgrLe1
      settings: AttributesFormatString=%<Priority>
  Data Store Write : DataStoreWrite  Priority=2  DataStoreName=UgrLe2
      settings: AttributesFormatString=%<Priority>
  Data Store Write1 : DataStoreWrite  Priority=2  DataStoreName=UgrLe1
      settings: AttributesFormatString=%<Priority>
  Product1 : Product  SaturateOnIntegerOverflow=on  InputSameDT=on
  Product2 : Product  SaturateOnIntegerOverflow=on
  Product3 : Product  SaturateOnIntegerOverflow=on
  Sum : Sum  Inputs=+-+
  Sum1 : Sum  Inputs=|++
  Sum2 : Sum  Inputs=|+-
  Filt : Outport
  wires:
  Sum2/1 -> Filt/1
  [a2] -> Product2/1
  Product2/1 -> Sum/2
  Product1/1 -> Sum/3
  [minus_a1] -> Product1/2
  Sum/1 -> Data Store Write1/1, Sum2/1
  Sum1/1 -> Product2/2
  Product3/1 -> Sum1/1, Sum/1
  a2/1 -> [a2]
  minus_a1/1 -> [minus_a1]
  y/1 -> [y]
  Constant3/1 -> Product3/2
  [y] -> Product3/1
  Data Store Read1/1 -> Data Store Write/1, Product1/1
  Data Store Read/1 -> [UgrLe2]
  [UgrLe2] -> Sum1/2
  [UgrLe2] -> Sum2/2

== system SF015A_WhlImbRejctn/WhlImbRejctn/WhlImbRejctnPer1/Whl Spd filter and Freq Estimation/UGR R/Calc_ma1_a2 ==
  note: Limit f_est to first and last
      | value in t_FreqScaleTblX
  f_est : Inport
  PoleMag : Inport  Port=2
  Add : Sum  Inputs=+-
  Constant1 : Constant
  Constant2 : Constant  Value=WhlImbRejctnFrqScaTblX
  Constant3 : Constant  Value=TWO_ULS_F32  OutDataTypeStr=single
  Constant4 : Constant  Value=WhlImbRejctnFrqScaTblX
  Constant5 : Constant  Value=0
  CopyRight2 : Subsystem  Description=|  mask(Copyright Information){none=on}
      | Copyright info block.                                               
      |                                                                     
      | Place copyright information at the top of every subsystem in design.
      mask prompts: none "No parameters"
      mask help: Place copyright information at the top of every subsystem in design.
      mask Display:
      | NxtrConf = 'Nexteer Confidential';
      | 
      | sys = bdroot; %handle for the current model ("system")
      | first = get_param(sys,'Created');
      | first = first(end-3:end);  %year is last four digits
      | 
      | last = get_param(sys,'LastModifiedDate');
      | if isempty(last)
      |     last = datestr(now,'yyyy');
      | else
      |     last = last(end-3:end);
      | end
      | 
      | if strcmp(first,last)
      |     fprintf('%s -- Copyright %s Nexteer',NxtrConf,first)
      | else
      |     fprintf('%s -- %s%s- %s Nexteer',NxtrConf,char(169),first,last)
      | end
  Cos_f32 : NxtrMath/Cos_f32  SFunctionSpec=single y1 = Cos_f32(single u1)
      settings: AttributesFormatString=%<MaskType>
  FixdToFloat_f32_u1 : FixdToFloat/FixdToFloat_f32_u16  Param1=0
  FixdToFloat_f32_u16 : FixdToFloat/FixdToFloat_f32_u16  Param1=0
  Gain : Gain  Gain=ARCHGLBPRM_2PI_ULS_F32
  LimDyn_f32 : NxtrLim/LimDyn_f32
  Math Function1 : Math  Operator=square  SaturateOnIntegerOverflow=on  OutDataTypeStr=Inherit: Inherit via internal rule
  Product1 : Product  Inputs=3  SaturateOnIntegerOverflow=on
  Product3 : Product  SaturateOnIntegerOverflow=on
  Selector3 : Selector  IndexMode=Zero-based  InputPortWidth=6  IndexOptions=Index vector (port)  Indices=[1]  OutputSizes=1
  Selector4 : Selector  IndexMode=Zero-based  InputPortWidth=6  IndexOptions=Index vector (port)  Indices=[1]  OutputSizes=1
  Ts : Constant  Value=ARCHGLBPRM_2MILLISEC_SEC_F32
  Width : Width
  minus_a1 : Outport
  a2 : Outport  Port=2
  wires:
  Gain/1 -> Cos_f32/1
  Product1/1 -> minus_a1/1  "ma1"
  Constant3/1 -> Product1/2
  Cos_f32/1 -> Product1/1
  Product3/1 -> Gain/1
  Ts/1 -> Product3/2
  PoleMag/1 -> Product1/3, Math Function1/1
  Math Function1/1 -> a2/1
  LimDyn_f32/1 -> Product3/1
  f_est/1 -> LimDyn_f32/1
  FixdToFloat_f32_u16/1 -> LimDyn_f32/3
  FixdToFloat_f32_u1/1 -> LimDyn_f32/2
  Selector3/1 -> FixdToFloat_f32_u16/1
  Selector4/1 -> FixdToFloat_f32_u1/1
  Constant4/1 -> Width/1, Selector3/1
  Constant5/1 -> Selector4/2
  Width/1 -> Add/1
  Add/1 -> Selector3/2
  Constant1/1 -> Add/2
  Constant2/1 -> Selector4/1

== system SF015A_WhlImbRejctn/WhlImbRejctn/WhlImbRejctnPer1/Whl Spd filter and Freq Estimation/UGR R/CopyRight2 ==

== system SF015A_WhlImbRejctn/WhlImbRejctn/WhlImbRejctnPer1/Whl Spd filter and Freq Estimation/UGR R/UnityGainResFilt ==
  y : Inport
  minus_a1 : Inport  Port=2
  a2 : Inport  Port=3
  Constant3 : Constant  Value=ONEHALF_ULS_F32
  CopyRight2 : Subsystem  Description=|  mask(Copyright Information){none=on}
      | Copyright info block.                                               
      |                                                                     
      | Place copyright information at the top of every subsystem in design.
      mask prompts: none "No parameters"
      mask help: Place copyright information at the top of every subsystem in design.
      mask Display:
      | NxtrConf = 'Nexteer Confidential';
      | 
      | sys = bdroot; %handle for the current model ("system")
      | first = get_param(sys,'Created');
      | first = first(end-3:end);  %year is last four digits
      | 
      | last = get_param(sys,'LastModifiedDate');
      | if isempty(last)
      |     last = datestr(now,'yyyy');
      | else
      |     last = last(end-3:end);
      | end
      | 
      | if strcmp(first,last)
      |     fprintf('%s -- Copyright %s Nexteer',NxtrConf,first)
      | else
      |     fprintf('%s -- %s%s- %s Nexteer',NxtrConf,char(169),first,last)
      | end
  Data Store Read2 : DataStoreRead  Priority=1  DataStoreName=UgrRi2
      settings: AttributesFormatString=%<Priority>
  Data Store Read3 : DataStoreRead  Priority=1  DataStoreName=UgrRi1
      settings: AttributesFormatString=%<Priority>
  Data Store Write : DataStoreWrite  Priority=2  DataStoreName=UgrRi2
      settings: AttributesFormatString=%<Priority>
  Data Store Write1 : DataStoreWrite  Priority=2  DataStoreName=UgrRi1
      settings: AttributesFormatString=%<Priority>
  Product1 : Product  SaturateOnIntegerOverflow=on  InputSameDT=on
  Product2 : Product  SaturateOnIntegerOverflow=on
  Product3 : Product  SaturateOnIntegerOverflow=on
  Sum : Sum  Inputs=+-+
  Sum1 : Sum  Inputs=|++
  Sum2 : Sum  Inputs=|+-
  Filt : Outport
  wires:
  Sum2/1 -> Filt/1
  [a2] -> Product2/1
  Product2/1 -> Sum/2
  Product1/1 -> Sum/3
  [minus_a1] -> Product1/2
  Sum/1 -> Data Store Write1/1, Sum2/1
  Sum1/1 -> Product2/2
  Product3/1 -> Sum1/1, Sum/1
  a2/1 -> [a2]
  minus_a1/1 -> [minus_a1]
  y/1 -> [y]
  Constant3/1 -> Product3/2
  [y] -> Product3/1
  Data Store Read2/1 -> [UgrRi2]
  Data Store Read3/1 -> Data Store Write/1, Product1/1
  [UgrRi2] -> Sum1/2
  [UgrRi2] -> Sum2/2

== system SF015A_WhlImbRejctn/WhlImbRejctn/WhlImbRejctnPer2/Flt Recovery- DC Trend/ElapsedTime1/CopyRight2 ==

== system SF015A_WhlImbRejctn/WhlImbRejctn/WhlImbRejctnPer2/Flt Recovery- DC Trend/ElapsedTime1/If not true elapsed time = 0 ==
  Action Port : ActionPort  ActionType=then
  Constant : Constant  Value=0  OutDataTypeStr=single
  CopyRight2 : Subsystem  Description=|  mask(Copyright Information){none=on}
      | Copyright info block.                                               
      |                                                                     
      | Place copyright information at the top of every subsystem in design.
      mask prompts: none "No parameters"
      mask help: Place copyright information at the top of every subsystem in design.
      mask Display:
      | NxtrConf = 'Nexteer Confidential';
      | 
      | sys = bdroot; %handle for the current model ("system")
      | first = get_param(sys,'Created');
      | first = first(end-3:end);  %year is last four digits
      | 
      | last = get_param(sys,'LastModifiedDate');
      | if isempty(last)
      |     last = datestr(now,'yyyy');
      | else
      |     last = last(end-3:end);
      | end
      | 
      | if strcmp(first,last)
      |     fprintf('%s -- Copyright %s Nexteer',NxtrConf,first)
      | else
      |     fprintf('%s -- %s%s- %s Nexteer',NxtrConf,char(169),first,last)
      | end
  SpanTi : Outport
  wires:
  Constant/1 -> SpanTi/1

== system SF015A_WhlImbRejctn/WhlImbRejctn/WhlImbRejctnPer2/Flt Recovery- DC Trend/ElapsedTime1/If true and last step is true calculate elapsed time  ==
  Action Port : ActionPort  ActionType=else
  Constant1 : Constant  Value=MICROSECTOMILLISEC_ULS_F32
  CopyRight2 : Subsystem  Description=|  mask(Copyright Information){none=on}
      | Copyright info block.                                               
      |                                                                     
      | Place copyright information at the top of every subsystem in design.
      mask prompts: none "No parameters"
      mask help: Place copyright information at the top of every subsystem in design.
      mask Display:
      | NxtrConf = 'Nexteer Confidential';
      | 
      | sys = bdroot; %handle for the current model ("system")
      | first = get_param(sys,'Created');
      | first = first(end-3:end);  %year is last four digits
      | 
      | last = get_param(sys,'LastModifiedDate');
      | if isempty(last)
      |     last = datestr(now,'yyyy');
      | else
      |     last = last(end-3:end);
      | end
      | 
      | if strcmp(first,last)
      |     fprintf('%s -- Copyright %s Nexteer',NxtrConf,first)
      | else
      |     fprintf('%s -- %s%s- %s Nexteer',NxtrConf,char(169),first,last)
      | end
  Data Store Read : DataStoreRead  DataStoreName=DcTrendRefTiEnaLrng
  Divide : Product  Inputs=**
  FixdToFloat_f32_u32 : FixdToFloat/FixdToFloat_f32_u32  Param1=0
  GetTiSpan100MicroSec32bit : Subsystem
  SpanTi : Outport
  wires:
  Constant1/1 -> Divide/2
  Divide/1 -> SpanTi/1
  GetTiSpan100MicroSec32bit/1(TiSpan) -> FixdToFloat_f32_u32/1
  Data Store Read/1 -> GetTiSpan100MicroSec32bit/1(RefTmr)
  FixdToFloat_f32_u32/1 -> Divide/1
